simulink model "TeamA_PAsqualo_R19b"  (R2019b)
settings: Solver=VariableStepAuto  StartTime=0.0  StopTime=stop_time  FixedStep=0.05  RelTol=1e-3
InitFcn:
  | main_init
values from neighbouring files (symbols this model uses):
  a1 = rho * D^4 * alpha1    (= 0.000388302366464)    [data_current.m]    (also in main_init.m)
  a2 = -rho * D^3 * alpha2 * (1 - omega)    (= 0.0037030698432)    [data_current.m]    (also in main_init.m)
  ag = [Ax Ay Az]'    [init_modello.m]
  alpha1 = 0.0113    [data_current.m]    (also in main_init.m)
  alpha2 = -0.0091    [data_current.m]    (also in main_init.m)
  areaOfInterestCorner = [42.317744;10.915136; 0]    [init_controllo.m]    (also in missionA.m = [42.317744)
  bg = [Bx By Bz]'    [init_modello.m]
  cd_pitch = 0.7    [init_modello.m]
  cd_roll = 0.04    [init_modello.m]
  cd_x = 0.4    [init_modello.m]
  cd_y = 1    [init_modello.m]
  cd_yaw = 0.7    [init_modello.m]
  cd_z = 1    [init_modello.m]
  cg = [Cx Cy Cz]'    [init_modello.m]
  D = 0.076    [data_current.m]    (also in main_init.m)
  dead_zone_limit = 31.5    [data_current.m]    (also in main_init.m)
  dg = [Dx Dy Dz]'    [init_modello.m]
  eg = [Ex Ey Ez]'    [init_modello.m]
  fg = [Fx Fy Fz]'    [init_modello.m]
  g = 9.81    [init_modello.m]
  galleggiamento = 66.5386    [init_controllo.m]
  gg = [Gx Gy Gz]'    [init_modello.m]
  H0 = 0    [init_modello.m]
  init_position = [pointP(1),pointP(2),0.15,0,0,deg2rad(angle)]'    [appunti.m]    (also in init_modello.m = [pointP(1),pointP(2),0.15,0,0,deg2rad(alpha)]')
  init_velocity = [0 0 0 0 0 0]'    [init_modello.m]
  initial_state_cov = blkdiag(diag(cov_gps(1,1:2)), cov_depth*eye(n_state_filter-2))    [init_navigazione.m]
  Ixx = 0.93304097392    [init_modello.m]
  Ixy = 0    [init_modello.m]
  Ixz = 0    [init_modello.m]
  Iyy = 25.58745481378    (= 25.5874548138)    [init_modello.m]
  Iyz = 0    [init_modello.m]
  Izz = 25.58745481378    (= 25.5874548138)    [init_modello.m]
  K_i_heave_div = 20    [init_controllo.m]
  K_i_heave_pos = 1    [init_controllo.m]
  K_i_heave_surf = 20    [init_controllo.m]
  K_i_heave_trans = 5    [init_controllo.m]
  K_i_heave_turn = 5    [init_controllo.m]
  K_i_pitch_div = 0    [init_controllo.m]
  K_i_pitch_pos = 0.1*0    (= 0)    [init_controllo.m]
  K_i_pitch_surf = 0    [init_controllo.m]
  K_i_pitch_trans = 0    [init_controllo.m]
  K_i_pitch_turn = 0    [init_controllo.m]
  K_i_roll_div = 0    [init_controllo.m]
  K_i_roll_pos = 0.1*0    (= 0)    [init_controllo.m]
  K_i_roll_surf = 1    [init_controllo.m]
  K_i_roll_trans = 0    [init_controllo.m]
  K_i_roll_turn = 0    [init_controllo.m]
  K_i_surge_div = 3    [init_controllo.m]
  K_i_surge_pos = 0.1679*30    (= 5.037)    [init_controllo.m]
  K_i_surge_surf = 3    [init_controllo.m]
  K_i_surge_trans = 0.1679*15    (= 2.5185)    [init_controllo.m]
  K_i_surge_turn = 0.1679*60    (= 10.074)    [init_controllo.m]
  K_i_sway_div = 6    [init_controllo.m]
  K_i_sway_pos = 5    [init_controllo.m]
  K_i_sway_surf = 3    [init_controllo.m]
  K_i_sway_trans = 2    [init_controllo.m]
  K_i_sway_turn = 50    [init_controllo.m]
  K_i_yaw_div = 0    [init_controllo.m]
  K_i_yaw_pos = 1    [init_controllo.m]
  K_i_yaw_surf = 0    [init_controllo.m]
  K_i_yaw_trans = 20    [init_controllo.m]
  K_p_heave_div = 200    [init_controllo.m]
  K_p_heave_pos = 320    [init_controllo.m]
  K_p_heave_surf = 200    [init_controllo.m]
  K_p_heave_trans = 170    [init_controllo.m]
  K_p_heave_turn = 170    [init_controllo.m]
  K_p_phi_div = 0.15    [init_controllo.m]
  K_p_phi_pos = 1*0.1    (= 0.1)    [init_controllo.m]
  K_p_phi_surf = 0.15    [init_controllo.m]
  K_p_phi_trans = 0.1    [init_controllo.m]
  K_p_phi_turn = 0.1    [init_controllo.m]
  K_p_pitch_div = 50    [init_controllo.m]
  K_p_pitch_pos = 25    [init_controllo.m]
  K_p_pitch_surf = 50    [init_controllo.m]
  K_p_pitch_trans = 25    [init_controllo.m]
  K_p_pitch_turn = 25    [init_controllo.m]
  K_p_psi_div = 0.3    [init_controllo.m]
  K_p_psi_pos = 0.25    [init_controllo.m]
  K_p_psi_surf = 0.3    [init_controllo.m]
  K_p_psi_trans = 0.2    [init_controllo.m]
  K_p_roll_div = 10    [init_controllo.m]
  K_p_roll_pos = 0.1*40    (= 4)    [init_controllo.m]
  K_p_roll_surf = 10    [init_controllo.m]
  K_p_roll_trans = 0.1*40    (= 4)    [init_controllo.m]
  K_p_roll_turn = 4    [init_controllo.m]
  K_p_surge_div = 80    [init_controllo.m]
  K_p_surge_pos = 13.7782*2.5    (= 34.4455)    [init_controllo.m]
  K_p_surge_surf = 80    [init_controllo.m]
  K_p_surge_trans = 20    [init_controllo.m]
  K_p_surge_turn = 150    [init_controllo.m]
  K_p_sway_div = 100    [init_controllo.m]
  K_p_sway_pos = 90    [init_controllo.m]
  K_p_sway_surf = 80    [init_controllo.m]
  K_p_sway_trans = 80    [init_controllo.m]
  K_p_sway_turn = 200    [init_controllo.m]
  K_p_th_div = 0.3    [init_controllo.m]
  K_p_th_pos = 0.1    [init_controllo.m]
  K_p_th_surf = 0.3    [init_controllo.m]
  K_p_th_trans = 0.1    [init_controllo.m]
  K_p_th_turn = 0.1    [init_controllo.m]
  K_p_x_div = 0.12    [init_controllo.m]
  K_p_x_pos = 0.12    [init_controllo.m]
  K_p_x_surf = 0.12    [init_controllo.m]
  K_p_y_div = 0.6    [init_controllo.m]
  K_p_y_pos = 0.34    [init_controllo.m]
  K_p_y_surf = 0.1    [init_controllo.m]
  K_p_y_trans = 0.3    [init_controllo.m]
  K_p_y_turn = 0.3    [init_controllo.m]
  K_p_yaw_div = 70    [init_controllo.m]
  K_p_yaw_pos = 20    [init_controllo.m]
  K_p_yaw_surf = 70    [init_controllo.m]
  K_p_yaw_trans = 160    [init_controllo.m]
  K_p_z_div = 0.35    [init_controllo.m]
  K_p_z_pos = 0.2    [init_controllo.m]
  K_p_z_surf = 0.35    [init_controllo.m]
  K_p_z_trans = 0.10    (= 0.1)    [init_controllo.m]
  K_p_z_turn = 0.1    [init_controllo.m]
  Kadd = 0    [init_modello.m]
  m = 100    [init_modello.m]    (also in retta.m = p2-p1)
  Madd = -((((1/5)*(b^2-a^2)^2))*(alpha_0-beta_0))/((((2*(b^2-a^2)^2))+(b^2-a^2)^2)*(alpha_0-beta_0)*m)    [init_modello.m]
  ... (+59 more)
undefined symbols (not defined in the file or in its folder): DiscIntNeverNeededParam, initial_state
libraries: simulink x2, vrlib x1
(part 2 of 6)

== system TeamA_PAsqualo_R19b/controller1/surfacing controller ==
  enable : Inport
  references : Inport  Port=2
  est_state : Inport  Port=3
  Mux : Mux  Inputs=6
  heave_controller : Subsystem
  pitch_controller : Subsystem
  roll_controller : Subsystem
  surge_controller : Subsystem
  sway_controller : Subsystem
  yaw_controller : Subsystem
  tau_surf : Outport
  wires:
  sway_controller/1(Y) -> Mux/2  "Y"
  yaw_controller/1(N) -> Mux/6  "N"
  Mux/1 -> tau_surf/1
  heave_controller/1(Z) -> Mux/3  "Z"
  references/1 -> surge_controller/2(references), heave_controller/2(references), roll_controller/2(references), yaw_controller/2(references), pitch_controller/2(references), sway_controller/2(references)
  est_state/1 -> sway_controller/3("estimated measures "), heave_controller/3("estimated measures "), roll_controller/3("estimated measures "), yaw_controller/3("estimated measures "), pitch_controller/3("estimated measures "), surge_controller/3("estimated measures ")
  surge_controller/1(X) -> Mux/1  "X"
  roll_controller/1(K) -> Mux/4  "K"
  pitch_controller/1(M) -> Mux/5  "M"
  enable/1 -> sway_controller/1(enable), heave_controller/1(enable), yaw_controller/1(enable), pitch_controller/1(enable), roll_controller/1(enable), surge_controller/1(enable)

== system TeamA_PAsqualo_R19b/controller1/transect controller ==
  enable : Inport
  references : Inport  Port=2
  est_state : Inport  Port=3
  Mux : Mux  Inputs=6
  heave_controller : Subsystem
  pitch_controller : Subsystem
  roll_controller : Subsystem
  surge_controller : Subsystem
  sway_controller : Subsystem
  yaw_controller : Subsystem
  tau_trans : Outport
  wires:
  sway_controller/1(Y) -> Mux/2  "Y"
  yaw_controller/1(N) -> Mux/6  "N"
  Mux/1 -> tau_trans/1
  heave_controller/1(Z) -> Mux/3  "Z"
  references/1 -> surge_controller/2(references), heave_controller/2(references), roll_controller/2(references), yaw_controller/2(references), pitch_controller/2(references), sway_controller/2(references)
  est_state/1 -> sway_controller/3("estimated measures "), heave_controller/3("estimated measures "), roll_controller/3("estimated measures "), yaw_controller/3("estimated measures "), pitch_controller/3("estimated measures "), surge_controller/3("estimated measures ")
  surge_controller/1(X) -> Mux/1  "X"
  roll_controller/1(K) -> Mux/4  "K"
  pitch_controller/1(M) -> Mux/5  "M"
  enable/1 -> sway_controller/1(enable), heave_controller/1(enable), yaw_controller/1(enable), pitch_controller/1(enable), roll_controller/1(enable), surge_controller/1(enable)

== system TeamA_PAsqualo_R19b/controller1/turning controller ==
  enable : Inport
  references : Inport  Port=2
  est_state : Inport  Port=3
  Mux : Mux  Inputs=6
  heave_controller : Subsystem
  pitch_controller : Subsystem
  roll_controller : Subsystem
  surge_controller : Subsystem
  sway_controller : Subsystem
  yaw_controller : Subsystem
  tau_turn : Outport
  wires:
  sway_controller/1(Y) -> Mux/2  "Y"
  yaw_controller/1(N) -> Mux/6  "N"
  Mux/1 -> tau_turn/1
  heave_controller/1(Z) -> Mux/3  "Z"
  references/1 -> surge_controller/2(references), heave_controller/2(references), roll_controller/2(references), yaw_controller/2(references), pitch_controller/2(references), sway_controller/2(references)
  est_state/1 -> sway_controller/3("estimated measures "), heave_controller/3("estimated measures "), roll_controller/3("estimated measures "), yaw_controller/3("estimated measures "), pitch_controller/3("estimated measures "), surge_controller/3("estimated measures ")
  surge_controller/1(X) -> Mux/1  "X"
  roll_controller/1(K) -> Mux/4  "K"
  pitch_controller/1(M) -> Mux/5  "M"
  enable/1 -> sway_controller/1(enable), heave_controller/1(enable), yaw_controller/1(enable), pitch_controller/1(enable), roll_controller/1(enable), surge_controller/1(enable)

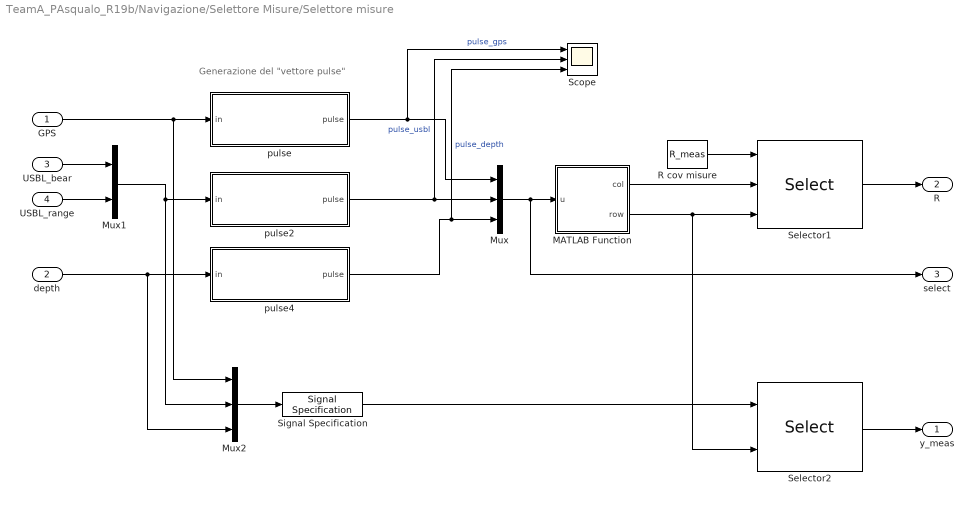
== system TeamA_PAsqualo_R19b/Navigazione/Selettore Misure/Selettore misure ==
  note: Generazione del "vettore pulse"
  GPS : Inport
  depth : Inport  Port=2
  USBL_bear : Inport  Port=3
  USBL_range : Inport  Port=4
  MATLAB Function : MATLAB Function  TreatAsAtomicUnit=on
  Mux : Mux  Inputs=3
  Mux1 : Mux  Inputs=2
  Mux2 : Mux  Inputs=3
  R cov misure : Constant  Value=R_meas
  Scope : Scope  NumInputPorts=3
  Selector1 : Selector  NumberOfDimensions=2  InputPortWidth=3  IndexOptions=Index vector (port),Index vector (port)  Indices=[1 3],1  OutputSizes=1,1
  Selector2 : Selector  InputPortWidth=5  IndexOptions=Index vector (port)  Indices=[1 3]  OutputSizes=1
  Signal Specification : SignalSpecification  Dimensions=[5 1]
  pulse : Subsystem
  pulse2 : Subsystem
  pulse4 : Subsystem
  y_meas : Outport
  R : Outport  Port=2
  select : Outport  Port=3
  wires:
  MATLAB Function/2(row) -> Selector1/3, Selector2/2
  Mux/1 -> select/1, MATLAB Function/1(u)
  R cov misure/1 -> Selector1/1
  MATLAB Function/1(col) -> Selector1/2
  pulse4/1(pulse) -> Scope/3, Mux/3  "pulse_depth"
  pulse/1(pulse) -> Scope/1, Mux/1  "pulse_gps"
  pulse2/1(pulse) -> Mux/2, Scope/2  "pulse_usbl"
  USBL_bear/1 -> Mux1/1
  USBL_range/1 -> Mux1/2
  Selector1/1 -> R/1
  Mux2/1 -> Signal Specification/1
  Selector2/1 -> y_meas/1
  GPS/1 -> Mux2/1, pulse/1(in)
  Mux1/1 -> pulse2/1(in), Mux2/2
  depth/1 -> Mux2/3, pulse4/1(in)
  Signal Specification/1 -> Selector2/1

== system TeamA_PAsqualo_R19b/controller1/diving controller/heave_controller ==
  enable : Inport
  references : Inport  Port=2
  "estimated measures " : Inport  Port=3
  Heave PID controller : Subsystem
  Z : Outport
  wires:
  Heave PID controller/1(Z) -> Z/1  "Z_pid"
  references/1 -> Heave PID controller/2(references)
  enable/1 -> Heave PID controller/1(enable)
  "estimated measures "/1 -> Heave PID controller/3("estimated measures ")

== system TeamA_PAsqualo_R19b/controller1/diving controller/pitch_controller ==
  enable : Inport
  references : Inport  Port=2
  "estimated measures " : Inport  Port=3
  Pitch PID controller : Subsystem
  M : Outport
  wires:
  enable/1 -> Pitch PID controller/1(enable)
  "estimated measures "/1 -> Pitch PID controller/3("estimated measures ")
  references/1 -> Pitch PID controller/2(references)
  Pitch PID controller/1(tau_pitch) -> M/1  "M_pid"

== system TeamA_PAsqualo_R19b/controller1/diving controller/roll_controller ==
  enable : Inport
  references : Inport  Port=2
  "estimated measures " : Inport  Port=3
  Roll PID controller : Subsystem
  K : Outport
  wires:
  "estimated measures "/1 -> Roll PID controller/3("estimated measures ")
  Roll PID controller/1(tau_roll) -> K/1  "K_pid"
  references/1 -> Roll PID controller/2(references)
  enable/1 -> Roll PID controller/1(enable)

== system TeamA_PAsqualo_R19b/controller1/diving controller/surge_controller ==
  enable : Inport
  references : Inport  Port=2
  "estimated measures " : Inport  Port=3
  Surge PID controller : Subsystem
  X : Outport
  wires:
  references/1 -> Surge PID controller/2(references)
  "estimated measures "/1 -> Surge PID controller/3("estimated measures ")
  Surge PID controller/1(X) -> X/1  "X_pid"
  enable/1 -> Surge PID controller/1(enable)

== system TeamA_PAsqualo_R19b/controller1/diving controller/sway_controller ==
  enable : Inport
  references : Inport  Port=2
  "estimated measures " : Inport  Port=3
  Sway PID controller : Subsystem
  Y : Outport
  wires:
  enable/1 -> Sway PID controller/1(enable)
  "estimated measures "/1 -> Sway PID controller/3("estimated measures ")
  references/1 -> Sway PID controller/2(references)
  Sway PID controller/1(Y) -> Y/1  "Y_pid"

== system TeamA_PAsqualo_R19b/controller1/diving controller/yaw_controller ==
  enable : Inport
  references : Inport  Port=2
  "estimated measures " : Inport  Port=3
  Yaw PID controller : Subsystem
  N : Outport
  wires:
  enable/1 -> Yaw PID controller/1(enable)
  "estimated measures "/1 -> Yaw PID controller/3("estimated measures ")
  references/1 -> Yaw PID controller/2(references)
  Yaw PID controller/1(tau_yaw) -> N/1  "N_pid"

== system TeamA_PAsqualo_R19b/controller1/positioning controller/heave_controller ==
  enable : Inport
  references : Inport  Port=2
  "estimated measures " : Inport  Port=3
  Heave PID controller : Subsystem
  Z : Outport
  wires:
  Heave PID controller/1(Z) -> Z/1  "Z_pid"
  references/1 -> Heave PID controller/2(references)  "ref"
  enable/1 -> Heave PID controller/1(enable)
  "estimated measures "/1 -> Heave PID controller/3("estimated measures ")  "est_meas"

== system TeamA_PAsqualo_R19b/controller1/positioning controller/pitch_controller ==
  enable : Inport
  references : Inport  Port=2
  "estimated measures " : Inport  Port=3
  Pitch PID controller : Subsystem
  M : Outport
  wires:
  enable/1 -> Pitch PID controller/1(enable)
  "estimated measures "/1 -> Pitch PID controller/3("estimated measures ")
  references/1 -> Pitch PID controller/2(references)
  Pitch PID controller/1(tau_pitch) -> M/1  "M_pid"

== system TeamA_PAsqualo_R19b/controller1/positioning controller/roll_controller ==
  enable : Inport
  references : Inport  Port=2
  "estimated measures " : Inport  Port=3
  Roll PID controller : Subsystem
  K : Outport
  wires:
  "estimated measures "/1 -> Roll PID controller/3("estimated measures ")
  Roll PID controller/1(tau_roll) -> K/1  "K_pid"
  references/1 -> Roll PID controller/2(references)
  enable/1 -> Roll PID controller/1(enable)

== system TeamA_PAsqualo_R19b/controller1/positioning controller/surge_controller ==
  enable : Inport
  references : Inport  Port=2
  "estimated measures " : Inport  Port=3
  Surge PID controller : Subsystem
  X : Outport
  wires:
  references/1 -> Surge PID controller/2(references)  "ref"
  "estimated measures "/1 -> Surge PID controller/3("estimated measures ")  "est_meas"
  Surge PID controller/1(X) -> X/1  "X_pid"
  enable/1 -> Surge PID controller/1(enable)

== system TeamA_PAsqualo_R19b/controller1/positioning controller/sway_controller ==
  enable : Inport
  references : Inport  Port=2
  "estimated measures " : Inport  Port=3
  Sway PID controller : Subsystem
  Y : Outport
  wires:
  enable/1 -> Sway PID controller/1(enable)
  "estimated measures "/1 -> Sway PID controller/3("estimated measures ")
  references/1 -> Sway PID controller/2(references)
  Sway PID controller/1(Y) -> Y/1  "Y_pid"

== system TeamA_PAsqualo_R19b/controller1/positioning controller/yaw_controller ==
  enable : Inport
  references : Inport  Port=2
  "estimated measures " : Inport  Port=3
  Yaw PID controller : Subsystem
  N : Outport
  wires:
  enable/1 -> Yaw PID controller/1(enable)
  "estimated measures "/1 -> Yaw PID controller/3("estimated measures ")  "est_meas"
  references/1 -> Yaw PID controller/2(references)  "ref"
  Yaw PID controller/1(tau_yaw) -> N/1  "N_pid"

== system TeamA_PAsqualo_R19b/controller1/surfacing controller/heave_controller ==
  enable : Inport
  references : Inport  Port=2
  "estimated measures " : Inport  Port=3
  Heave PID controller : Subsystem
  Z : Outport
  wires:
  Heave PID controller/1(Z) -> Z/1  "Z_pid"
  references/1 -> Heave PID controller/2(references)
  enable/1 -> Heave PID controller/1(enable)
  "estimated measures "/1 -> Heave PID controller/3("estimated measures ")

== system TeamA_PAsqualo_R19b/controller1/surfacing controller/pitch_controller ==
  enable : Inport
  references : Inport  Port=2
  "estimated measures " : Inport  Port=3
  Pitch PID controller : Subsystem
  M : Outport
  wires:
  enable/1 -> Pitch PID controller/1(enable)
  "estimated measures "/1 -> Pitch PID controller/3("estimated measures ")
  references/1 -> Pitch PID controller/2(references)
  Pitch PID controller/1(M) -> M/1  "M_pid"

== system TeamA_PAsqualo_R19b/controller1/surfacing controller/roll_controller ==
  enable : Inport
  references : Inport  Port=2
  "estimated measures " : Inport  Port=3
  Roll PID controller : Subsystem
  K : Outport
  wires:
  "estimated measures "/1 -> Roll PID controller/3("estimated measures ")
  Roll PID controller/1(K) -> K/1  "K_pid"
  references/1 -> Roll PID controller/2(references)
  enable/1 -> Roll PID controller/1(enable)

== system TeamA_PAsqualo_R19b/controller1/surfacing controller/surge_controller ==
  enable : Inport
  references : Inport  Port=2
  "estimated measures " : Inport  Port=3
  Surge PID controller : Subsystem
  X : Outport
  wires:
  references/1 -> Surge PID controller/2(references)
  "estimated measures "/1 -> Surge PID controller/3("estimated measures ")
  Surge PID controller/1(X) -> X/1  "X_pid"
  enable/1 -> Surge PID controller/1(enable)

== system TeamA_PAsqualo_R19b/controller1/surfacing controller/sway_controller ==
  enable : Inport
  references : Inport  Port=2
  "estimated measures " : Inport  Port=3
  Sway PID controller : Subsystem
  Y : Outport
  wires:
  enable/1 -> Sway PID controller/1(enable)
  "estimated measures "/1 -> Sway PID controller/3("estimated measures ")
  references/1 -> Sway PID controller/2(references)
  Sway PID controller/1(Y) -> Y/1  "Y_pid"

== system TeamA_PAsqualo_R19b/controller1/surfacing controller/yaw_controller ==
  enable : Inport
  references : Inport  Port=2
  "estimated measures " : Inport  Port=3
  Yaw PID controller : Subsystem
  N : Outport
  wires:
  enable/1 -> Yaw PID controller/1(enable)
  "estimated measures "/1 -> Yaw PID controller/3("estimated measures ")
  references/1 -> Yaw PID controller/2(references)
  Yaw PID controller/1(N) -> N/1  "N_pid"

== system TeamA_PAsqualo_R19b/controller1/transect controller/heave_controller ==
  enable : Inport
  references : Inport  Port=2
  "estimated measures " : Inport  Port=3
  Heave PID controller : Subsystem
  Z : Outport
  wires:
  Heave PID controller/1(Z) -> Z/1  "Z_pid"
  references/1 -> Heave PID controller/2(references)
  enable/1 -> Heave PID controller/1(enable)
  "estimated measures "/1 -> Heave PID controller/3("estimated measures ")

== system TeamA_PAsqualo_R19b/controller1/transect controller/pitch_controller ==
  enable : Inport
  references : Inport  Port=2
  "estimated measures " : Inport  Port=3
  Pitch PID controller : Subsystem
  M : Outport
  wires:
  enable/1 -> Pitch PID controller/1(enable)
  "estimated measures "/1 -> Pitch PID controller/3("estimated measures ")
  references/1 -> Pitch PID controller/2(references)
  Pitch PID controller/1(M) -> M/1  "M_pid"

== system TeamA_PAsqualo_R19b/controller1/transect controller/roll_controller ==
  enable : Inport
  references : Inport  Port=2
  "estimated measures " : Inport  Port=3
  Roll PID controller : Subsystem
  K : Outport
  wires:
  "estimated measures "/1 -> Roll PID controller/3("estimated measures ")
  Roll PID controller/1(tau_roll) -> K/1  "K_pid"
  references/1 -> Roll PID controller/2(references)
  enable/1 -> Roll PID controller/1(enable)

== system TeamA_PAsqualo_R19b/controller1/transect controller/surge_controller ==
  enable : Inport
  references : Inport  Port=2
  "estimated measures " : Inport  Port=3
  Surge PID controller : Subsystem
  X : Outport
  wires:
  references/1 -> Surge PID controller/2(ref)
  "estimated measures "/1 -> Surge PID controller/3(est_meas)
  Surge PID controller/1(X) -> X/1  "X_pid"
  enable/1 -> Surge PID controller/1(enable)

== system TeamA_PAsqualo_R19b/controller1/transect controller/sway_controller ==
  enable : Inport
  references : Inport  Port=2
  "estimated measures " : Inport  Port=3
  Sway PID controller : Subsystem
  Y : Outport
  wires:
  enable/1 -> Sway PID controller/1(enable)
  "estimated measures "/1 -> Sway PID controller/3("estimated measures ")
  references/1 -> Sway PID controller/2(references)
  Sway PID controller/1(Y) -> Y/1  "Y_pid"

== system TeamA_PAsqualo_R19b/controller1/transect controller/yaw_controller ==
  enable : Inport
  references : Inport  Port=2
  "estimated measures " : Inport  Port=3
  Yaw PID controller : Subsystem
  N : Outport
  wires:
  enable/1 -> Yaw PID controller/1(enable)
  "estimated measures "/1 -> Yaw PID controller/3("estimated measures ")
  references/1 -> Yaw PID controller/2(references)
  Yaw PID controller/1(N) -> N/1  "N_pid"

== system TeamA_PAsqualo_R19b/controller1/turning controller/heave_controller ==
  enable : Inport
  references : Inport  Port=2
  "estimated measures " : Inport  Port=3
  Heave PID controller : Subsystem
  Z : Outport
  wires:
  Heave PID controller/1(Z) -> Z/1  "Z_pid"
  references/1 -> Heave PID controller/2(references)
  enable/1 -> Heave PID controller/1(enable)
  "estimated measures "/1 -> Heave PID controller/3("estimated measures ")

== system TeamA_PAsqualo_R19b/controller1/turning controller/pitch_controller ==
  enable : Inport
  references : Inport  Port=2
  "estimated measures " : Inport  Port=3
  Pitch PID controller : Subsystem
  M : Outport
  wires:
  enable/1 -> Pitch PID controller/1(enable)
  "estimated measures "/1 -> Pitch PID controller/3("estimated measures ")
  references/1 -> Pitch PID controller/2(references)
  Pitch PID controller/1(M) -> M/1  "M_pid"

== system TeamA_PAsqualo_R19b/controller1/turning controller/roll_controller ==
  enable : Inport
  references : Inport  Port=2
  "estimated measures " : Inport  Port=3
  Roll PID controller : Subsystem
  K : Outport
  wires:
  "estimated measures "/1 -> Roll PID controller/3("estimated measures ")
  Roll PID controller/1(K) -> K/1  "K_pid"
  references/1 -> Roll PID controller/2(references)
  enable/1 -> Roll PID controller/1(enable)

== system TeamA_PAsqualo_R19b/controller1/turning controller/surge_controller ==
  enable : Inport
  references : Inport  Port=2
  "estimated measures " : Inport  Port=3
  Surge PID controller : Subsystem
  X : Outport
  wires:
  references/1 -> Surge PID controller/2(ref)
  "estimated measures "/1 -> Surge PID controller/3(est_meas)
  Surge PID controller/1(X) -> X/1  "X_pid"
  enable/1 -> Surge PID controller/1(enable)

== system TeamA_PAsqualo_R19b/controller1/turning controller/sway_controller ==
  enable : Inport
  references : Inport  Port=2
  "estimated measures " : Inport  Port=3
  Sway PID controller : Subsystem
  Y : Outport
  wires:
  enable/1 -> Sway PID controller/1(enable)
  "estimated measures "/1 -> Sway PID controller/3("estimated measures ")
  references/1 -> Sway PID controller/2(references)
  Sway PID controller/1(Y) -> Y/1  "Y_pid"

== system TeamA_PAsqualo_R19b/controller1/turning controller/yaw_controller ==
  enable : Inport
  references : Inport  Port=2
  "estimated measures " : Inport  Port=3
  Yaw PID controller : Subsystem
  N : Outport
  wires:
  enable/1 -> Yaw PID controller/1(enable)
  "estimated measures "/1 -> Yaw PID controller/3(est_meas)
  references/1 -> Yaw PID controller/2(ref)
  Yaw PID controller/1(N) -> N/1  "N_pid"

== system TeamA_PAsqualo_R19b/Navigazione/Selettore Misure/Selettore misure/pulse ==
  in : Inport
  Delay : Delay  DelayLength=1  SampleTime=ts_filter
  MATLAB Function : MATLAB Function  TreatAsAtomicUnit=on
  Scope : Scope
  Scope1 : Scope
  Sum2 : Sum  Inputs=|+-
  pulse : Outport
  wires:
  Sum2/1 -> MATLAB Function/2(u)
  in/1 -> Scope1/1, Delay/1, Sum2/1, MATLAB Function/1(gps_now)
  Delay/1 -> Sum2/2
  MATLAB Function/1(y) -> Scope/1, pulse/1

== system TeamA_PAsqualo_R19b/Navigazione/Selettore Misure/Selettore misure/pulse2 ==
  in : Inport
  Delay : Delay  DelayLength=1  SampleTime=ts_filter
  MATLAB Function : MATLAB Function  TreatAsAtomicUnit=on
  Sum2 : Sum  Inputs=|+-
  pulse : Outport
  wires:
  Sum2/1 -> MATLAB Function/1(u)
  in/1 -> Delay/1, Sum2/1
  Delay/1 -> Sum2/2
  MATLAB Function/1(y) -> pulse/1

== system TeamA_PAsqualo_R19b/Navigazione/Selettore Misure/Selettore misure/pulse4 ==
  in : Inport
  Delay : Delay  DelayLength=1  SampleTime=ts_filter
  MATLAB Function : MATLAB Function  TreatAsAtomicUnit=on
  Sum2 : Sum  Inputs=|+-
  pulse : Outport
  wires:
  Sum2/1 -> MATLAB Function/1(u)
  in/1 -> Delay/1, Sum2/1
  Delay/1 -> Sum2/2
  MATLAB Function/1(y) -> pulse/1

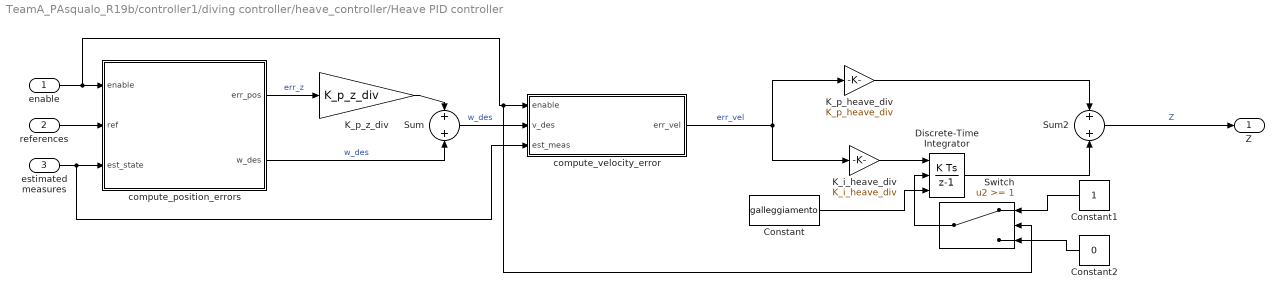
== system TeamA_PAsqualo_R19b/controller1/diving controller/heave_controller/Heave PID controller ==
  enable : Inport
  references : Inport  Port=2
  "estimated measures " : Inport  Port=3
  Constant : Constant  Value=galleggiamento
  Constant1 : Constant
  Constant2 : Constant  Value=0
  Discrete-Time Integrator : DiscreteIntegrator  ExternalReset=falling  InitialConditionSource=external  SampleTime=0.1  ICPrevOutput=DiscIntNeverNeededParam  ICPrevScaledInput=DiscIntNeverNeededParam
  K_i_heave_div : Gain  Gain=K_i_heave_div
  K_p_heave_div : Gain  Gain=K_p_heave_div
  K_p_z_div : Gain  Gain=K_p_z_div
  Sum : Sum
  Sum2 : Sum
  Switch : Switch  Threshold=1
  compute_position_errors : MATLAB Function  TreatAsAtomicUnit=on
  compute_velocity_error : MATLAB Function  TreatAsAtomicUnit=on
  Z : Outport
  wires:
  "estimated measures "/1 -> compute_velocity_error/3(est_meas), compute_position_errors/3(est_state)
  K_p_z_div/1 -> Sum/1
  compute_position_errors/1(err_pos) -> K_p_z_div/1  "err_z"
  references/1 -> compute_position_errors/2(ref)
  Sum/1 -> compute_velocity_error/2(v_des)  "w_des"
  compute_position_errors/2(w_des) -> Sum/2  "w_des"
  K_p_heave_div/1 -> Sum2/1
  K_i_heave_div/1 -> Discrete-Time Integrator/1
  compute_velocity_error/1(err_vel) -> K_i_heave_div/1, K_p_heave_div/1  "err_vel"
  Sum2/1 -> Z/1  "Z"
  Discrete-Time Integrator/1 -> Sum2/2
  Constant/1 -> Discrete-Time Integrator/3
  Switch/1 -> Discrete-Time Integrator/2
  enable/1 -> Switch/2, compute_velocity_error/1(enable), compute_position_errors/1(enable)
  Constant2/1 -> Switch/3
  Constant1/1 -> Switch/1

== system TeamA_PAsqualo_R19b/controller1/diving controller/pitch_controller/Pitch PID controller ==
  enable : Inport
  references : Inport  Port=2
  "estimated measures " : Inport  Port=3
  Constant : Constant
  Constant1 : Constant  Value=0
  Discrete-Time Integrator : DiscreteIntegrator  ExternalReset=falling  SampleTime=0.1  ICPrevOutput=DiscIntNeverNeededParam  ICPrevScaledInput=DiscIntNeverNeededParam
  K_i_pitch_div : Gain  Gain=K_i_pitch_div
  K_p_pitch_div : Gain  Gain=K_p_pitch_div
  K_p_th_div : Gain  Gain=K_p_th_div
  Sum2 : Sum
  Switch : Switch  Threshold=1
  compute_orientation_errors : MATLAB Function  TreatAsAtomicUnit=on
  compute_velocity_error : MATLAB Function  TreatAsAtomicUnit=on
  tau_pitch : Outport
  wires:
  references/1 -> compute_orientation_errors/2(ref)
  K_p_th_div/1 -> compute_velocity_error/2(v_des)
  "estimated measures "/1 -> compute_velocity_error/3(est_meas), compute_orientation_errors/3(est_state)
  compute_orientation_errors/1(err_orient) -> K_p_th_div/1  "err_orient"
  K_p_pitch_div/1 -> Sum2/1
  Sum2/1 -> tau_pitch/1  "tau_pitch"
  K_i_pitch_div/1 -> Discrete-Time Integrator/1
  Discrete-Time Integrator/1 -> Sum2/2
  compute_velocity_error/1(err_vel) -> K_i_pitch_div/1, K_p_pitch_div/1  "err_vel"
  Switch/1 -> Discrete-Time Integrator/2
  enable/1 -> Switch/2, compute_velocity_error/1(enable), compute_orientation_errors/1(enable)
  Constant1/1 -> Switch/3
  Constant/1 -> Switch/1

== system TeamA_PAsqualo_R19b/controller1/diving controller/roll_controller/Roll PID controller ==
  enable : Inport
  references : Inport  Port=2
  "estimated measures " : Inport  Port=3
  Constant : Constant
  Constant1 : Constant  Value=0
  Discrete-Time Integrator : DiscreteIntegrator  ExternalReset=falling  SampleTime=0.1  ICPrevOutput=DiscIntNeverNeededParam  ICPrevScaledInput=DiscIntNeverNeededParam
  K_i_roll_div : Gain  Gain=K_i_roll_div
  K_p_phi_div : Gain  Gain=K_p_phi_div
  K_p_roll_div : Gain  Gain=K_p_roll_div
  Sum2 : Sum
  Switch : Switch  Threshold=1
  compute_orientation_errors : MATLAB Function  TreatAsAtomicUnit=on
  compute_velocity_error : MATLAB Function  TreatAsAtomicUnit=on
  tau_roll : Outport
  wires:
  "estimated measures "/1 -> compute_velocity_error/3(est_meas), compute_orientation_errors/3(est_state)
  K_p_phi_div/1 -> compute_velocity_error/2(v_des)
  compute_orientation_errors/1(err_orient) -> K_p_phi_div/1  "err_orient"
  references/1 -> compute_orientation_errors/2(ref)
  K_p_roll_div/1 -> Sum2/1
  Sum2/1 -> tau_roll/1  "tau_roll"
  K_i_roll_div/1 -> Discrete-Time Integrator/1
  Discrete-Time Integrator/1 -> Sum2/2
  compute_velocity_error/1(err_vel) -> K_i_roll_div/1, K_p_roll_div/1  "err_vel"
  Switch/1 -> Discrete-Time Integrator/2
  enable/1 -> Switch/2, compute_velocity_error/1(enable), compute_orientation_errors/1(enable)
  Constant1/1 -> Switch/3
  Constant/1 -> Switch/1

== system TeamA_PAsqualo_R19b/controller1/diving controller/surge_controller/Surge PID controller ==
  enable : Inport
  references : Inport  Port=2
  "estimated measures " : Inport  Port=3
  Constant : Constant
  Constant1 : Constant  Value=0
  Discrete-Time Integrator : DiscreteIntegrator  ExternalReset=falling  SampleTime=0.1  ICPrevOutput=DiscIntNeverNeededParam  ICPrevScaledInput=DiscIntNeverNeededParam
  K_i_surge_div : Gain  Gain=K_i_surge_div
  K_p_surge_div : Gain  Gain=K_p_surge_div
  K_p_x_div : Gain  Gain=K_p_x_div
  Sum2 : Sum
  Switch : Switch  Threshold=1
  compute_position_errors : MATLAB Function  TreatAsAtomicUnit=on
  compute_velocity_error : MATLAB Function  TreatAsAtomicUnit=on
  X : Outport
  wires:
  references/1 -> compute_position_errors/2(ref)
  compute_position_errors/1(err_pos) -> K_p_x_div/1  "err_x"
  "estimated measures "/1 -> compute_velocity_error/3(est_meas), compute_position_errors/3(est_state)
  K_p_x_div/1 -> compute_velocity_error/2(v_des)
  Sum2/1 -> X/1  "X"
  K_p_surge_div/1 -> Sum2/1
  Discrete-Time Integrator/1 -> Sum2/2
  K_i_surge_div/1 -> Discrete-Time Integrator/1
  compute_velocity_error/1(err_vel) -> K_i_surge_div/1, K_p_surge_div/1  "err_vel"
  Switch/1 -> Discrete-Time Integrator/2
  enable/1 -> Switch/2, compute_velocity_error/1(enable), compute_position_errors/1(enable)
  Constant1/1 -> Switch/3
  Constant/1 -> Switch/1

== system TeamA_PAsqualo_R19b/controller1/diving controller/sway_controller/Sway PID controller ==
  enable : Inport
  references : Inport  Port=2
  "estimated measures " : Inport  Port=3
  Constant : Constant
  Constant1 : Constant  Value=0
  Discrete-Time Integrator : DiscreteIntegrator  ExternalReset=falling  SampleTime=0.1  ICPrevOutput=DiscIntNeverNeededParam  ICPrevScaledInput=DiscIntNeverNeededParam
  K_i_sway_div : Gain  Gain=K_i_sway_div
  K_p_sway_div : Gain  Gain=K_p_sway_div
  K_p_y_div : Gain  Gain=K_p_y_div
  Sum2 : Sum
  Switch : Switch  Threshold=1
  compute_position_errors : MATLAB Function  TreatAsAtomicUnit=on
  compute_velocity_error : MATLAB Function  TreatAsAtomicUnit=on
  Y : Outport
  wires:
  references/1 -> compute_position_errors/2(ref)
  compute_position_errors/1(err_pos) -> K_p_y_div/1  "err_y"
  K_p_y_div/1 -> compute_velocity_error/2(v_des)  "v_des_sway"
  "estimated measures "/1 -> compute_velocity_error/3(est_meas), compute_position_errors/3(est_state)
  K_p_sway_div/1 -> Sum2/1
  Sum2/1 -> Y/1  "Y"
  K_i_sway_div/1 -> Discrete-Time Integrator/1
  Discrete-Time Integrator/1 -> Sum2/2
  compute_velocity_error/1(err_vel) -> K_i_sway_div/1, K_p_sway_div/1  "err_vel"
  Switch/1 -> Discrete-Time Integrator/2
  enable/1 -> Switch/2, compute_velocity_error/1(enable), compute_position_errors/1(enable)
  Constant1/1 -> Switch/3
  Constant/1 -> Switch/1

== system TeamA_PAsqualo_R19b/controller1/diving controller/yaw_controller/Yaw PID controller ==
  enable : Inport
  references : Inport  Port=2
  "estimated measures " : Inport  Port=3
  Constant : Constant
  Constant1 : Constant  Value=0
  Discrete-Time Integrator : DiscreteIntegrator  ExternalReset=falling  SampleTime=0.1  ICPrevOutput=DiscIntNeverNeededParam  ICPrevScaledInput=DiscIntNeverNeededParam
  K_i_yaw_div : Gain  Gain=K_i_yaw_div
  K_p_psi_div : Gain  Gain=K_p_psi_div
  K_p_yaw_div : Gain  Gain=K_p_yaw_div
  Sum2 : Sum
  Switch : Switch  Threshold=1
  compute_orientation_errors : MATLAB Function  TreatAsAtomicUnit=on
  compute_velocity_error : MATLAB Function  TreatAsAtomicUnit=on
  tau_yaw : Outport
  wires:
  references/1 -> compute_orientation_errors/2(ref)
  "estimated measures "/1 -> compute_velocity_error/3(est_meas), compute_orientation_errors/3(est_state)
  compute_orientation_errors/1(err_orient) -> K_p_psi_div/1  "err_orient"
  K_p_psi_div/1 -> compute_velocity_error/2(v_des)
  K_p_yaw_div/1 -> Sum2/1
  Sum2/1 -> tau_yaw/1  "tau_yaw"
  K_i_yaw_div/1 -> Discrete-Time Integrator/1
  Discrete-Time Integrator/1 -> Sum2/2
  compute_velocity_error/1(err_vel) -> K_i_yaw_div/1, K_p_yaw_div/1  "err_vel"
  Switch/1 -> Discrete-Time Integrator/2
  enable/1 -> compute_velocity_error/1(enable), Switch/2, compute_orientation_errors/1(enable)
  Constant1/1 -> Switch/3
  Constant/1 -> Switch/1

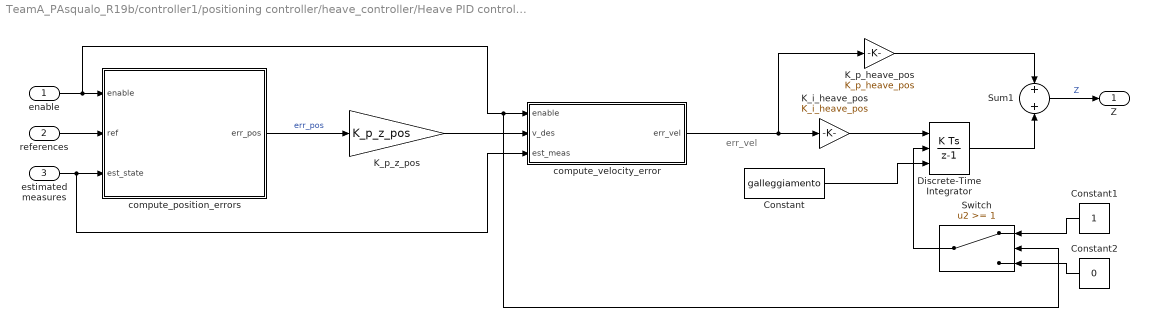
== system TeamA_PAsqualo_R19b/controller1/positioning controller/heave_controller/Heave PID controller ==
  note: err_vel
  enable : Inport
  references : Inport  Port=2
  "estimated measures " : Inport  Port=3
  Constant : Constant  Value=galleggiamento
  Constant1 : Constant
  Constant2 : Constant  Value=0
  Discrete-Time Integrator : DiscreteIntegrator  ExternalReset=falling  InitialConditionSource=external  SampleTime=0.1  ICPrevOutput=DiscIntNeverNeededParam  ICPrevScaledInput=DiscIntNeverNeededParam
  K_i_heave_pos : Gain  Gain=K_i_heave_pos
  K_p_heave_pos : Gain  Gain=K_p_heave_pos
  K_p_z_pos : Gain  Gain=K_p_z_pos
  Sum1 : Sum
  Switch : Switch  Threshold=1
  compute_position_errors : MATLAB Function  TreatAsAtomicUnit=on
  compute_velocity_error : MATLAB Function  TreatAsAtomicUnit=on
  Z : Outport
  wires:
  "estimated measures "/1 -> compute_velocity_error/3(est_meas), compute_position_errors/3(est_state)
  K_p_z_pos/1 -> compute_velocity_error/2(v_des)
  compute_position_errors/1(err_pos) -> K_p_z_pos/1  "err_pos"
  references/1 -> compute_position_errors/2(ref)
  K_i_heave_pos/1 -> Discrete-Time Integrator/1
  compute_velocity_error/1(err_vel) -> K_i_heave_pos/1, K_p_heave_pos/1
  K_p_heave_pos/1 -> Sum1/1
  Discrete-Time Integrator/1 -> Sum1/2
  Sum1/1 -> Z/1  "Z"
  Constant/1 -> Discrete-Time Integrator/3
  Switch/1 -> Discrete-Time Integrator/2
  enable/1 -> compute_velocity_error/1(enable), Switch/2, compute_position_errors/1(enable)
  Constant2/1 -> Switch/3
  Constant1/1 -> Switch/1

== system TeamA_PAsqualo_R19b/controller1/positioning controller/pitch_controller/Pitch PID controller ==
  enable : Inport
  references : Inport  Port=2
  "estimated measures " : Inport  Port=3
  Constant : Constant
  Constant1 : Constant  Value=0
  Discrete-Time Integrator : DiscreteIntegrator  ExternalReset=falling  SampleTime=0.1  ICPrevOutput=DiscIntNeverNeededParam  ICPrevScaledInput=DiscIntNeverNeededParam
  K_i_pitch_pos : Gain  Gain=K_i_pitch_pos
  K_p_pitch_pos : Gain  Gain=K_p_pitch_pos
  K_p_th_pos : Gain  Gain=K_p_th_pos
  Sum1 : Sum
  Switch : Switch  Threshold=1
  compute_orientation_errors : MATLAB Function  TreatAsAtomicUnit=on
  compute_velocity_error : MATLAB Function  TreatAsAtomicUnit=on
  tau_pitch : Outport
  wires:
  references/1 -> compute_orientation_errors/2(ref)
  K_p_th_pos/1 -> compute_velocity_error/2(v_des)
  Sum1/1 -> tau_pitch/1  "tau_pitch"
  "estimated measures "/1 -> compute_velocity_error/3(est_meas), compute_orientation_errors/3(est_state)
  compute_orientation_errors/1(err_orient) -> K_p_th_pos/1  "err_orient"
  K_i_pitch_pos/1 -> Discrete-Time Integrator/1
  compute_velocity_error/1(err_vel) -> K_i_pitch_pos/1, K_p_pitch_pos/1  "err_vel"
  Discrete-Time Integrator/1 -> Sum1/2
  K_p_pitch_pos/1 -> Sum1/1
  Switch/1 -> Discrete-Time Integrator/2
  enable/1 -> Switch/2, compute_velocity_error/1(enable), compute_orientation_errors/1(enable)
  Constant1/1 -> Switch/3
  Constant/1 -> Switch/1

== system TeamA_PAsqualo_R19b/controller1/positioning controller/roll_controller/Roll PID controller ==
  note: err_vel
  enable : Inport
  references : Inport  Port=2
  "estimated measures " : Inport  Port=3
  Constant : Constant
  Constant1 : Constant  Value=0
  Discrete-Time Integrator : DiscreteIntegrator  ExternalReset=falling  SampleTime=0.1  ICPrevOutput=DiscIntNeverNeededParam  ICPrevScaledInput=DiscIntNeverNeededParam
  K_i_roll_pos : Gain  Gain=K_i_roll_pos
  K_p_phi_pos : Gain  Gain=K_p_phi_pos
  K_p_roll_pos : Gain  Gain=K_p_roll_pos
  Sum1 : Sum
  Switch : Switch  Threshold=1
  compute_orientation_errors : MATLAB Function  TreatAsAtomicUnit=on
  compute_velocity_error : MATLAB Function  TreatAsAtomicUnit=on
  tau_roll : Outport
  wires:
  "estimated measures "/1 -> compute_velocity_error/3(est_meas), compute_orientation_errors/3(est_state)
  Sum1/1 -> tau_roll/1  "tau_roll"
  K_p_phi_pos/1 -> compute_velocity_error/2(v_des)  "v_des"
  compute_orientation_errors/1(err_orient) -> K_p_phi_pos/1  "err_orient"
  references/1 -> compute_orientation_errors/2(ref)
  K_i_roll_pos/1 -> Discrete-Time Integrator/1
  compute_velocity_error/1(err_vel) -> K_i_roll_pos/1, K_p_roll_pos/1
  Discrete-Time Integrator/1 -> Sum1/2
  K_p_roll_pos/1 -> Sum1/1
  Switch/1 -> Discrete-Time Integrator/2
  enable/1 -> Switch/2, compute_velocity_error/1(enable), compute_orientation_errors/1(enable)
  Constant1/1 -> Switch/3
  Constant/1 -> Switch/1

== system TeamA_PAsqualo_R19b/controller1/positioning controller/surge_controller/Surge PID controller ==
  enable : Inport
  references : Inport  Port=2
  "estimated measures " : Inport  Port=3
  Constant3 : Constant
  Constant4 : Constant  Value=0
  Discrete-Time Integrator1 : DiscreteIntegrator  ExternalReset=falling  SampleTime=0.1  ICPrevOutput=DiscIntNeverNeededParam  ICPrevScaledInput=DiscIntNeverNeededParam
  K_i_surge_pos : Gain  Gain=K_i_surge_pos
  K_p_surge_pos : Gain  Gain=K_p_surge_pos
  K_p_x_pos : Gain  Gain=K_p_x_pos
  Sum : Sum
  Sum2 : Sum
  Switch1 : Switch  Threshold=1
  compute_position_errors : MATLAB Function  TreatAsAtomicUnit=on
  compute_velocity_error : MATLAB Function  TreatAsAtomicUnit=on
  X : Outport
  wires:
  Constant3/1 -> Switch1/1
  Constant4/1 -> Switch1/3
  compute_position_errors/1(err_pos) -> K_p_x_pos/1
  K_i_surge_pos/1 -> Discrete-Time Integrator1/1
  Switch1/1 -> Discrete-Time Integrator1/2
  compute_position_errors/2(u_des) -> Sum/2  "u_des"
  Sum/1 -> compute_velocity_error/2(v_des)  "u_des"
  Sum2/1 -> X/1
  K_p_surge_pos/1 -> Sum2/1
  compute_velocity_error/1(err_vel) -> K_i_surge_pos/1, K_p_surge_pos/1  "err_vel"
  "estimated measures "/1 -> compute_velocity_error/3(est_meas), compute_position_errors/3(est_state)
  references/1 -> compute_position_errors/2(ref)
  K_p_x_pos/1 -> Sum/1
  enable/1 -> Switch1/2, compute_velocity_error/1(enable), compute_position_errors/1(enable)
  Discrete-Time Integrator1/1 -> Sum2/2

== system TeamA_PAsqualo_R19b/controller1/positioning controller/sway_controller/Sway PID controller ==
  enable : Inport
  references : Inport  Port=2
  "estimated measures " : Inport  Port=3
  Constant : Constant
  Constant1 : Constant  Value=0
  Discrete-Time Integrator : DiscreteIntegrator  ExternalReset=falling  SampleTime=0.1  ICPrevOutput=DiscIntNeverNeededParam  ICPrevScaledInput=DiscIntNeverNeededParam
  K_i_sway_pos : Gain  Gain=K_i_sway_pos
  K_p_sway_pos : Gain  Gain=K_p_sway_pos
  K_p_y_pos : Gain  Gain=K_p_y_pos
  Sum1 : Sum
  Switch : Switch  Threshold=1
  compute_position_errors : MATLAB Function  TreatAsAtomicUnit=on
  compute_velocity_error : MATLAB Function  TreatAsAtomicUnit=on
  Y : Outport
  wires:
  references/1 -> compute_position_errors/2(ref)
  K_p_y_pos/1 -> compute_velocity_error/2(v_des)
  "estimated measures "/1 -> compute_velocity_error/3(est_meas), compute_position_errors/3(est_state)
  K_i_sway_pos/1 -> Discrete-Time Integrator/1
  compute_velocity_error/1(err_vel) -> K_i_sway_pos/1, K_p_sway_pos/1  "err_vel"
  Discrete-Time Integrator/1 -> Sum1/2
  K_p_sway_pos/1 -> Sum1/1
  Sum1/1 -> Y/1  "Y"
  compute_position_errors/1(err_pos) -> K_p_y_pos/1  "err_y"
  Switch/1 -> Discrete-Time Integrator/2
  enable/1 -> Switch/2, compute_velocity_error/1(enable), compute_position_errors/1(enable)
  Constant1/1 -> Switch/3
  Constant/1 -> Switch/1

== system TeamA_PAsqualo_R19b/controller1/positioning controller/yaw_controller/Yaw PID controller ==
  enable : Inport
  references : Inport  Port=2
  "estimated measures " : Inport  Port=3
  Constant : Constant
  Constant1 : Constant  Value=0
  Discrete-Time Integrator : DiscreteIntegrator  ExternalReset=falling  SampleTime=0.1  ICPrevOutput=DiscIntNeverNeededParam  ICPrevScaledInput=DiscIntNeverNeededParam
  K_i_yaw_pos : Gain  Gain=K_i_yaw_pos
  K_p_psi_pos : Gain  Gain=K_p_psi_pos
  K_p_yaw_pos : Gain  Gain=K_p_yaw_pos
  Sum1 : Sum
  Switch : Switch  Threshold=1
  compute_orientation_errors : MATLAB Function  TreatAsAtomicUnit=on
  compute_velocity_error : MATLAB Function  TreatAsAtomicUnit=on
  tau_yaw : Outport
  wires:
  references/1 -> compute_orientation_errors/2(ref)
  Sum1/1 -> tau_yaw/1  "tau_yaw"
  "estimated measures "/1 -> compute_velocity_error/3(est_meas), compute_orientation_errors/3(est_state)
  compute_orientation_errors/1(err_orient) -> K_p_psi_pos/1  "err_orient"
  K_p_psi_pos/1 -> compute_velocity_error/2(v_des)
  K_i_yaw_pos/1 -> Discrete-Time Integrator/1
  compute_velocity_error/1(err_vel) -> K_i_yaw_pos/1, K_p_yaw_pos/1  "err_vel"
  Discrete-Time Integrator/1 -> Sum1/2
  K_p_yaw_pos/1 -> Sum1/1
  Switch/1 -> Discrete-Time Integrator/2
  enable/1 -> Switch/2, compute_velocity_error/1(enable), compute_orientation_errors/1(enable)
  Constant1/1 -> Switch/3
  Constant/1 -> Switch/1

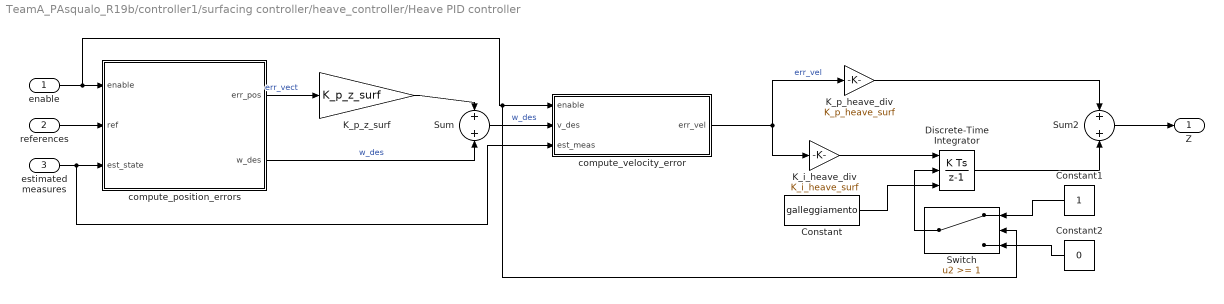
== system TeamA_PAsqualo_R19b/controller1/surfacing controller/heave_controller/Heave PID controller ==
  enable : Inport
  references : Inport  Port=2
  "estimated measures " : Inport  Port=3
  Constant : Constant  Value=galleggiamento
  Constant1 : Constant
  Constant2 : Constant  Value=0
  Discrete-Time Integrator : DiscreteIntegrator  ExternalReset=falling  InitialConditionSource=external  SampleTime=0.1  ICPrevOutput=DiscIntNeverNeededParam  ICPrevScaledInput=DiscIntNeverNeededParam
  K_i_heave_div : Gain  Gain=K_i_heave_surf
  K_p_heave_div : Gain  Gain=K_p_heave_surf
  K_p_z_surf : Gain  Gain=K_p_z_surf
  Sum : Sum
  Sum2 : Sum
  Switch : Switch  Threshold=1
  compute_position_errors : MATLAB Function  TreatAsAtomicUnit=on
  compute_velocity_error : MATLAB Function  TreatAsAtomicUnit=on
  Z : Outport
  wires:
  K_i_heave_div/1 -> Discrete-Time Integrator/1
  K_p_heave_div/1 -> Sum2/1
  references/1 -> compute_position_errors/2(ref)
  "estimated measures "/1 -> compute_velocity_error/3(est_meas), compute_position_errors/3(est_state)
  Sum/1 -> compute_velocity_error/2(v_des)  "w_des"
  compute_position_errors/1(err_pos) -> K_p_z_surf/1  "err_vect"
  compute_position_errors/2(w_des) -> Sum/2  "w_des"
  Sum2/1 -> Z/1
  K_p_z_surf/1 -> Sum/1
  compute_velocity_error/1(err_vel) -> K_i_heave_div/1, K_p_heave_div/1  "err_vel"
  Discrete-Time Integrator/1 -> Sum2/2
  Constant/1 -> Discrete-Time Integrator/3
  Switch/1 -> Discrete-Time Integrator/2
  enable/1 -> Switch/2, compute_velocity_error/1(enable), compute_position_errors/1(enable)
  Constant2/1 -> Switch/3
  Constant1/1 -> Switch/1

== system TeamA_PAsqualo_R19b/controller1/surfacing controller/pitch_controller/Pitch PID controller ==
  enable : Inport
  references : Inport  Port=2
  "estimated measures " : Inport  Port=3
  Constant : Constant
  Constant1 : Constant  Value=0
  Discrete-Time Integrator : DiscreteIntegrator  ExternalReset=falling  SampleTime=0.1  ICPrevOutput=DiscIntNeverNeededParam  ICPrevScaledInput=DiscIntNeverNeededParam
  K_i_pitch_surf : Gain  Gain=K_i_pitch_surf
  K_p_pitch_surf : Gain  Gain=K_p_pitch_surf
  K_p_th_surf : Gain  Gain=K_p_th_surf
  Sum2 : Sum
  Switch : Switch  Threshold=1
  compute_orientation_errors : MATLAB Function  TreatAsAtomicUnit=on
  compute_velocity_error : MATLAB Function  TreatAsAtomicUnit=on
  M : Outport
  wires:
  references/1 -> compute_orientation_errors/2(ref)
  K_p_th_surf/1 -> compute_velocity_error/2(v_des)
  "estimated measures "/1 -> compute_velocity_error/3(est_meas), compute_orientation_errors/3(est_state)
  compute_orientation_errors/1(err_orient) -> K_p_th_surf/1  "err_orient"
  Sum2/1 -> M/1
  Discrete-Time Integrator/1 -> Sum2/2
  K_i_pitch_surf/1 -> Discrete-Time Integrator/1
  K_p_pitch_surf/1 -> Sum2/1
  compute_velocity_error/1(err_vel) -> K_i_pitch_surf/1, K_p_pitch_surf/1  "err_vel"
  Switch/1 -> Discrete-Time Integrator/2
  enable/1 -> Switch/2, compute_velocity_error/1(enable), compute_orientation_errors/1(enable)
  Constant1/1 -> Switch/3
  Constant/1 -> Switch/1

== system TeamA_PAsqualo_R19b/controller1/surfacing controller/roll_controller/Roll PID controller ==
  enable : Inport
  references : Inport  Port=2
  "estimated measures " : Inport  Port=3
  Constant : Constant
  Constant1 : Constant  Value=0
  Discrete-Time Integrator : DiscreteIntegrator  ExternalReset=falling  SampleTime=0.1  ICPrevOutput=DiscIntNeverNeededParam  ICPrevScaledInput=DiscIntNeverNeededParam
  K_i_roll_surf : Gain  Gain=K_i_roll_surf
  K_p_phi_surf : Gain  Gain=K_p_phi_surf
  K_p_roll_surf : Gain  Gain=K_p_roll_surf
  Sum2 : Sum
  Switch : Switch  Threshold=1
  compute_orientation_errors : MATLAB Function  TreatAsAtomicUnit=on
  compute_velocity_error : MATLAB Function  TreatAsAtomicUnit=on
  K : Outport
  wires:
  "estimated measures "/1 -> compute_velocity_error/3(est_meas), compute_orientation_errors/3(est_state)
  K_p_phi_surf/1 -> compute_velocity_error/2(v_des)
  compute_orientation_errors/1(err_orient) -> K_p_phi_surf/1  "err_orient"
  references/1 -> compute_orientation_errors/2(ref)
  Sum2/1 -> K/1
  Discrete-Time Integrator/1 -> Sum2/2
  K_i_roll_surf/1 -> Discrete-Time Integrator/1
  K_p_roll_surf/1 -> Sum2/1
  compute_velocity_error/1(err_vel) -> K_i_roll_surf/1, K_p_roll_surf/1  "err_vel"
  Switch/1 -> Discrete-Time Integrator/2
  enable/1 -> Switch/2, compute_velocity_error/1(enable), compute_orientation_errors/1(enable)
  Constant1/1 -> Switch/3
  Constant/1 -> Switch/1

== system TeamA_PAsqualo_R19b/controller1/surfacing controller/surge_controller/Surge PID controller ==
  enable : Inport
  references : Inport  Port=2
  "estimated measures " : Inport  Port=3
  Constant : Constant
  Constant1 : Constant  Value=0
  Discrete-Time Integrator : DiscreteIntegrator  ExternalReset=falling  SampleTime=0.1  ICPrevOutput=DiscIntNeverNeededParam  ICPrevScaledInput=DiscIntNeverNeededParam
  K_i_surge_surf : Gain  Gain=K_i_surge_surf
  K_p_surge_surf : Gain  Gain=K_p_surge_surf
  K_p_x_surf : Gain  Gain=K_p_x_surf
  Sum2 : Sum
  Switch : Switch  Threshold=1
  compute_position_errors : MATLAB Function  TreatAsAtomicUnit=on
  compute_velocity_error : MATLAB Function  TreatAsAtomicUnit=on
  X : Outport
  wires:
  references/1 -> compute_position_errors/2(ref)
  compute_position_errors/1(err_pos) -> K_p_x_surf/1  "err_vect"
  K_p_x_surf/1 -> compute_velocity_error/2(v_des)
  "estimated measures "/1 -> compute_velocity_error/3(est_meas), compute_position_errors/3(est_state)
  K_i_surge_surf/1 -> Discrete-Time Integrator/1
  K_p_surge_surf/1 -> Sum2/1
  Sum2/1 -> X/1
  compute_velocity_error/1(err_vel) -> K_i_surge_surf/1, K_p_surge_surf/1  "err_vel"
  Discrete-Time Integrator/1 -> Sum2/2
  Switch/1 -> Discrete-Time Integrator/2
  enable/1 -> Switch/2, compute_velocity_error/1(enable), compute_position_errors/1(enable)
  Constant1/1 -> Switch/3
  Constant/1 -> Switch/1
